simulink model "modelisation2"  (R2016b)
settings: Solver=VariableStepAuto  StartTime=0.0  StopTime=20  MaxStep=0.01  RelTol=1e-3
settings Model: Creator=BOUDOT  LastModifiedBy=BOUDOT

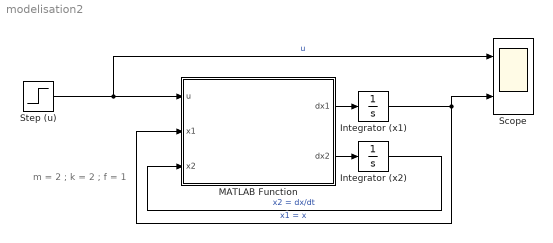
== system modelisation2 ==
  note: m = 2 ; k = 2 ; f = 1
  Integrator (x1) : Integrator
  Integrator (x2) : Integrator
  MATLAB Function : MATLAB Function  TreatAsAtomicUnit=on
  Scope : Scope  NumInputPorts=2
  Step (u) : Step  SampleTime=0
  wires:
  Step (u)/1 -> MATLAB Function/1(u), Scope/1  "u"
  MATLAB Function/1(dx1) -> Integrator (x1)/1
  MATLAB Function/2(dx2) -> Integrator (x2)/1
  Integrator (x2)/1 -> MATLAB Function/3(x2)  "x2 = dx/dt"
  Integrator (x1)/1 -> MATLAB Function/2(x1), Scope/2  "x1 = x"

== matlab function modelisation2/MATLAB Function ==
  data: u input; dx1 output; x1 input; x2 input; dx2 output
function [dx1, dx2] = system(u, x1, x2)

m = 2;
k = 2;
f = 1;

dx1 = x2;
dx2 = -k/m*x1 - f/m*x2 + 1/m*u;
